simulink model "estados"  (R2023a)
settings: Solver=VariableStepAuto  StartTime=0.0  StopTime=3  RelTol=1e-3
values from neighbouring files (symbols this model uses):
  A = [0 1; -k/m -b/m]    [estados.m]
  B = [0; 1/m]    [estados.m]
  h = double(kras.h(1))    [estados.m]
  k1 = double(kras.k1(1))    [estados.m]
  k2 = double(kras.k2(1))    [estados.m]
settings Model: Creator=a2270170  LastModifiedBy=a2270170

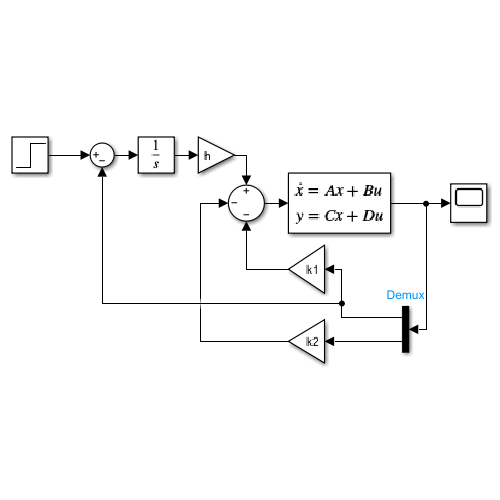
[thumbnail: Simulink's stored preview of the top-level diagram]
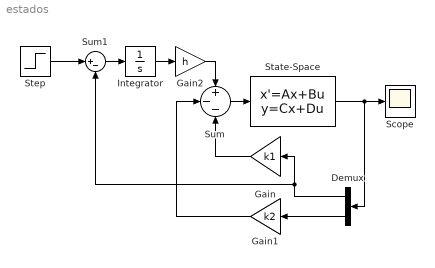
== system estados ==
  Demux : Demux  Outputs=2
  Gain : Gain  Gain=k1
  Gain1 : Gain  Gain=k2
  Gain2 : Gain  Gain=h
  Integrator : Integrator
  Scope : Scope
  State-Space : StateSpace  A=A  B=B  C=eye(2)  D=[0;0]  InitialCondition=0
  Step : Step  After=10  SampleTime=0
  Sum : Sum  Inputs=+--
  Sum1 : Sum  Inputs=|+-
  wires:
  State-Space/1 -> Scope/1, Demux/1
  Demux/2 -> Gain1/1
  Demux/1 -> Sum1/2, Gain/1
  Gain/1 -> Sum/3
  Gain1/1 -> Sum/2
  Sum/1 -> State-Space/1
  Integrator/1 -> Gain2/1
  Sum1/1 -> Integrator/1
  Gain2/1 -> Sum/1
  Step/1 -> Sum1/1
